simulink model "lidar_webcam_xyz"  (Simulink 7.3)
settings: Solver=FixedStepDiscrete  StartTime=0.0  StopTime=inf  MaxStep=0.2  RelTol=1e-3
settings Model: Creator=gclayton  LastModifiedBy=wildcat
settings DebuggingCC: InheritedTsInSrcMsg=none
settings RTWCC: SystemTargetFile=rlnx.tlc  GenCodeOnly=on  TemplateMakefile=rlnx_ubuntu.tmf  Description=Linux Real-Time Target  ProcessScript=rlnx_make_rtw_hook
settings RTWCC: CustomInclude=|
  | /usr/local/include/opencv/
  | /usr/local/include/
settings CodeAppCC: GenerateComments=off  SimulinkBlockComments=off
settings STFCustomTargetCC: ModelReferenceCompliant=off  MatFileLogging=on  SystemTargetFile=rlnx.tlc
settings GRTTargetCC: ModelReferenceCompliant=off  ParMdlRefBuildCompliant=off  CompOptLevelCompliant=off
settings CustomProperty: DataType=string  Value=-lm -ldl /usr/local/lib/libopencv_highgui.so.2.4 /usr/local/lib/libopencv_core.so.2.4 /usr/local/lib/libopencv_imgproc.so.2.4 -lc_urg -lc_urg_connection -lc_urg_system -lphidget21
settings EnumStrPairs: String=PC

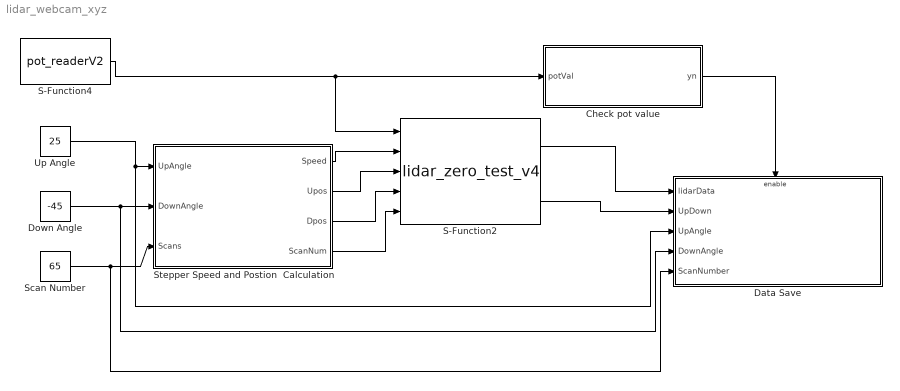
== system lidar_webcam_xyz ==
  Check pot value : Stateflow chart
  Data Save : Subsystem  TreatAsAtomicUnit=on
  Down Angle : Constant  Value=-45  OutDataType=fixdt(1, 16)  OutScaling=2^0
  S-Function2 : S-Function  FunctionName=lidar_zero_test_v4  EnableBusSupport=off
  S-Function4 : S-Function  FunctionName=pot_readerV2  EnableBusSupport=off
  Scan Number : Constant  Value=65  OutDataType=fixdt(1, 16)  OutScaling=2^0
  Stepper Speed and Postion  Calculation : Stateflow chart
  Up Angle : Constant  Value=25  OutDataType=fixdt(1, 16)  OutScaling=2^0
  wires:
  S-Function4/1 -> S-Function2/1, Check pot value/1(potVal)
  S-Function2/1 -> Data Save/1(lidarData)
  Check pot value/1(yn) -> Data Save/Enable
  Scan Number/1 -> Stepper Speed and Postion  Calculation/3(Scans), Data Save/5(ScanNumber)
  Down Angle/1 -> Stepper Speed and Postion  Calculation/2(DownAngle), Data Save/4(DownAngle)
  Up Angle/1 -> Data Save/3(UpAngle), Stepper Speed and Postion  Calculation/1(UpAngle)
  Stepper Speed and Postion  Calculation/1(Speed) -> S-Function2/2
  Stepper Speed and Postion  Calculation/2(Upos) -> S-Function2/3
  Stepper Speed and Postion  Calculation/3(Dpos) -> S-Function2/4
  Stepper Speed and Postion  Calculation/4(ScanNum) -> S-Function2/5
  S-Function2/2 -> Data Save/2(UpDown)

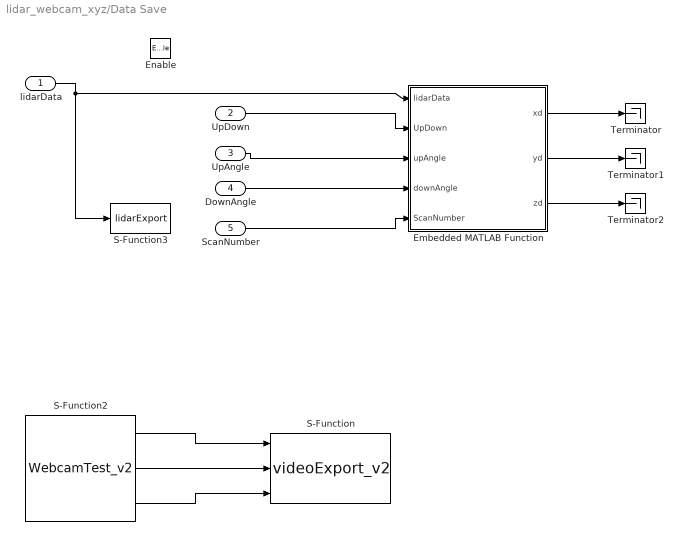
== system lidar_webcam_xyz/Data Save ==
  lidarData : Inport  OutDataType=fixdt(1, 16)  OutScaling=2^0
  UpDown : Inport  Port=2  OutDataType=fixdt(1, 16)  OutScaling=2^0
  UpAngle : Inport  Port=3  OutDataType=fixdt(1, 16)  OutScaling=2^0
  DownAngle : Inport  Port=4  OutDataType=fixdt(1, 16)  OutScaling=2^0
  ScanNumber : Inport  Port=5  OutDataType=fixdt(1, 16)  OutScaling=2^0
  Enable : EnablePort
  Embedded MATLAB Function : Stateflow chart
  S-Function : S-Function  FunctionName=videoExport_v2  EnableBusSupport=off
  S-Function2 : S-Function  FunctionName=WebcamTest_v2  EnableBusSupport=off
  S-Function3 : S-Function  FunctionName=lidarExport  EnableBusSupport=off
  Terminator : Terminator
  Terminator1 : Terminator
  Terminator2 : Terminator
  wires:
  S-Function2/3 -> S-Function/3
  S-Function2/2 -> S-Function/2
  S-Function2/1 -> S-Function/1
  lidarData/1 -> S-Function3/1, Embedded MATLAB Function/1(lidarData)
  UpDown/1 -> Embedded MATLAB Function/2(UpDown)
  UpAngle/1 -> Embedded MATLAB Function/3(upAngle)
  DownAngle/1 -> Embedded MATLAB Function/4(downAngle)
  ScanNumber/1 -> Embedded MATLAB Function/5(ScanNumber)
  Embedded MATLAB Function/3(zd) -> Terminator2/1
  Embedded MATLAB Function/2(yd) -> Terminator1/1
  Embedded MATLAB Function/1(xd) -> Terminator/1

== matlab function Check pot value ==
  data: potVal input double; yn output double
function yn = check_pot_val(potVal)
%#eml

% Pot value may initially be zero.
% Check for this and output a 1 or zero to 
% control whether the rest of model runs
if (potVal == 0)
    yn = 0;
else
    yn = 1;
end

== matlab function Data Save/Embedded MATLAB Function ==
  data: lidarData input double; xd output double; yd output double; zd output double; UpDown input double; upAngle input double; downAngle input double; ScanNumber input double
function [xd, yd, zd] = xyz_calc(lidarData,UpDown,upAngle,downAngle,ScanNumber)
%#eml

% Define variables based on gimbal system and scan pattern
ScanNum = ScanNumber;
DataLength = 1080*ScanNum;
h = 36.3;

% Define Data sizes
phim = zeros(1,DataLength);
thetam = zeros(1,DataLength);
distm = zeros(1,DataLength);
xd = zeros(1,DataLength);
yd = zeros(1,DataLength);
zd = zeros(1,DataLength);


%Define phi_rad: angles corresponding to one lidar scan
l = 1:1080;
phi_rad = (-45 + 0.25*l)*pi/180;

% Repeat thetam for number of scans
for i = 1:ScanNum
    % phi_start = 1+1080*(i-1);
    % phi_end = 1080*i;
    
    for j = 1 : 1080
        phi_val = 1080*(i-1) + j;
        phim(1,phi_val) = phi_rad(1,j);
    end
    % phim = [phim phi_rad]; 
end

% Calculate theta from the input angles
theta_min = downAngle*pi/180;
theta_max = upAngle*pi/180;
theta_step = (theta_max - theta_min)/DataLength;
if (UpDown == 0)
    % UpDown == 0, gimbal is moving down 
    thetam = [theta_max : -theta_step : (theta_min+theta_step)];
elseif (UpDown == 1)
    % UpDown == 1, gimbal is moving up
    thetam = [theta_min : theta_step : (theta_max-theta_step)];
end

% Distance matrix is directly obtained from lidar data
distm = lidarData';

% Calculate x y and z
for k = 1:DataLength
    % Replace returned zeros with large number
    if (distm(1,k) == 0)
        distm = 30000;
    end
    xd(1,k) = distm(1,k)*cos(phim(1,k));
    yd(1,k) = distm(1,k)*sin(phim(1,k))*cos(thetam(1,k)) - h*sin(thetam(1,k));
    zd(1,k) = distm(1,k)*sin(phim(1,k))*sin(thetam(1,k)) + h*cos(thetam(1,k));
end

== matlab function Stepper Speed and Postion Calculation ==
  data: UpAngle input double; Speed output double; DownAngle input double; Scans input double; Upos output double; Dpos output double; ScanNum output double
function [Speed,Upos,Dpos,ScanNum] = stepper_calc(UpAngle,DownAngle,Scans)

% This function inputs desired positive and negative scan angles
% and desired number of scans and outputs results positions for
% the stepper and the required speed of the stepper motor to properly
% move so the desired number of scans is obtained over the course of
% the motion of the stepper

% Scan Number requires no change
ScanNum = Scans;

% Transformation of angle to stepper position obtained from stepper calibration
% Output must be an integer
% 57 is added or subtracted due to wobble of gimbal system
Upos = round(UpAngle*1036/45)-57;
Dpos = round(DownAngle*1036/45)+57;

% Transformation of speed based 
% Output must be an interger
Speed = round(abs(UpAngle-DownAngle) * (1214/90) * 65/Scans);
